simulink model "bai3"  (R2018a)
settings: Solver=ode5  StartTime=0.0  StopTime=6  FixedStep=0.05  RelTol=1e-3
libraries: fuzblock x1
settings Model: Creator=trann  LastModifiedBy=DELL
settings SolverCC: AlgebraicLoopSolver=LineSearch

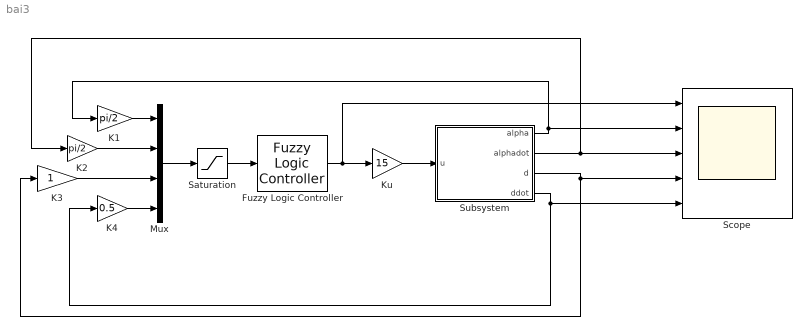
== system bai3 ==
  Fuzzy Logic Controller : fuzblock/Fuzzy Logic  Controller  FIS='fuzzy3.fis'  OutputSampleNumber=101  DataType=double  FuzzifiedInputs=off  RuleFiringStrengths=off  RuleOutputs=off  AggregatedOutputs=off  SimulateUsing=Interpreted execution  OutOfRangeInputValueMessage=warning  NoRuleFiredMessage=warning  EmptyOutputFuzzySetMessage=warning
  K1 : Gain  Gain=pi/2
  K2 : Gain  Gain=pi/2
  K3 : Gain
  K4 : Gain  Gain=0.5
  Ku : Gain  Gain=15
  Mux : Mux
  Saturation : Saturate  UpperLimit=1  LowerLimit=-1
  Scope : Scope  NumInputPorts=5
  Subsystem : Subsystem  mask{M1=3.3, m=0.49, g=9.81, a=0.11, c=0.045, J=0.42, km=5, b=5, d0=0.5, ddot0=-0.3, alpha0=-pi/6, alphadot0=pi/9}
      mask prompts: M1 "mass of balance"; m "mass of cart"; g "acceleration due to gravity"; a "height of track"; c "distance from center of gravity to point of rotation"; J "inertia of balance"; km "input-to-force gain"; b "damping coefficient"; d0 "vi tri dau"; ddot0 "van toc dau"; alpha0 "goc ban dau"; alphadot0 "van toc goc ban dau"
  wires:
  Ku/1 -> Subsystem/1(u)
  Mux/1 -> Saturation/1
  Saturation/1 -> Fuzzy Logic Controller/1
  Subsystem/1(alpha) -> K1/1, Scope/2
  Subsystem/2(alphadot) -> K2/1, Scope/3
  K1/1 -> Mux/1
  K2/1 -> Mux/2
  K3/1 -> Mux/3
  Subsystem/3(d) -> Scope/4, K3/1
  K4/1 -> Mux/4
  Subsystem/4(ddot) -> Scope/5, K4/1
  Fuzzy Logic Controller/1 -> Scope/1, Ku/1

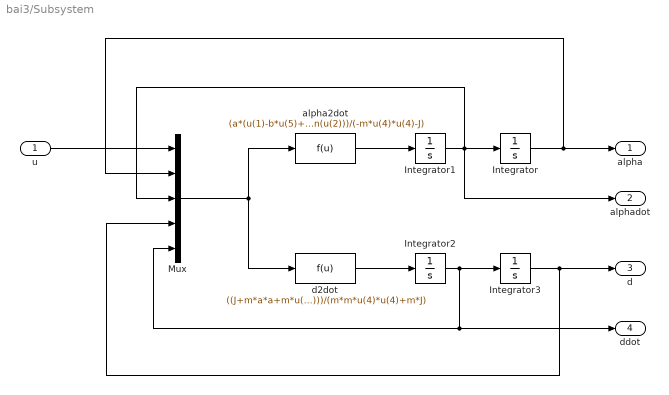
== system bai3/Subsystem ==
  u : Inport
  Integrator : Integrator  InitialCondition=alpha0
  Integrator1 : Integrator  InitialCondition=alphadot0
  Integrator2 : Integrator  InitialCondition=ddot0
  Integrator3 : Integrator  InitialCondition=d0
  Mux : Mux  Inputs=5
  alpha2dot : Fcn  Expr=(a*(u(1)-b*u(5)+m*u(4)*u(3)*u(3)+m*g*a*sin(u(2)))+2*u(3)*m*u(4)*u(5)-m*g*a*sin(u(2))-m*g*u(4)*cos(u(2))-M1*g*c*sin(u(2)))/(-m*u(4)*u(4)-J)
  d2dot : Fcn  Expr=((J+m*a*a+m*u(4)*u(4))*(km*u(1)-b*u(5)+m*u(4)*u(3)*u(3) +m*g*a*sin(u(2))) - m*a*(2*u(3)*m*u(4)*u(5)+m*g*a*sin(u(2))+m*g*u(4)*cos(u(2))+M1*g*c*sin(u(2))))/(m*m*u(4)*u(4)+m*J)
  alpha : Outport
  alphadot : Outport  Port=2
  d : Outport  Port=3
  ddot : Outport  Port=4
  wires:
  Integrator1/1 -> alphadot/1, Mux/3, Integrator/1
  Integrator/1 -> Mux/2, alpha/1
  alpha2dot/1 -> Integrator1/1
  Mux/1 -> d2dot/1, alpha2dot/1
  d2dot/1 -> Integrator2/1
  Integrator2/1 -> Mux/5, ddot/1, Integrator3/1
  Integrator3/1 -> Mux/4, d/1
  u/1 -> Mux/1
